simulink model "PLL_Sim_Rev0"  (R2019b)
settings: Solver=VariableStepAuto  StartTime=0.0  StopTime=0.0005  RelTol=1e-3
libraries: msbPllFoundation x1, impairlib x1, dspsrcs4 x1
settings Model: Creator=connerhannon  LastModifiedBy=connerhannon

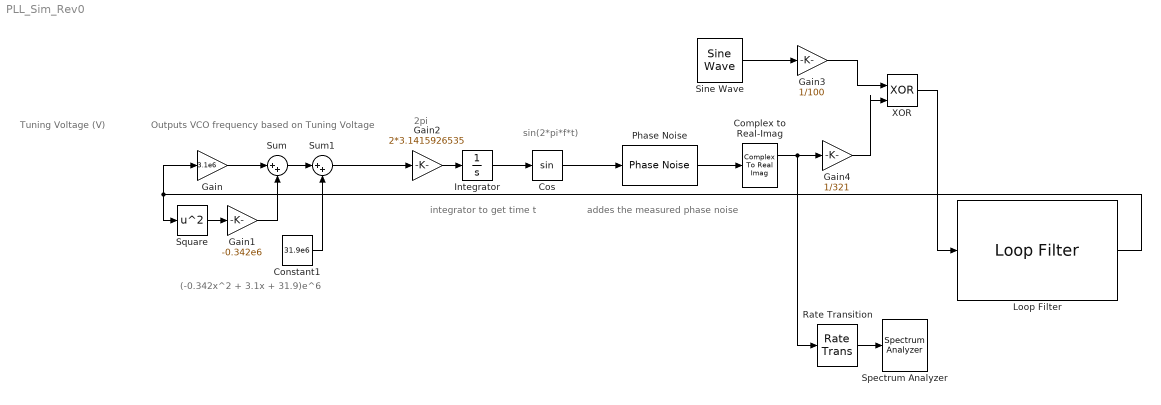
== system PLL_Sim_Rev0 ==
  note: Tuning Voltage
      | (V)
  note: 2pi
  note: sin(2*pi*f*t)
  note: integrator to get time t
  note: (-0.342x^2 + 3.1x + 31.9)e^6
  note: addes the measured phase noise
  note: Outputs VCO frequency based on Tuning Voltage
  Complex to Real-Imag : ComplexToRealImag
  Constant1 : Constant  Value=31.9e6
  Cos : Trigonometry  OutputSignalType=complex
  Gain : Gain  Gain=3.1e6
  Gain1 : Gain  Gain=-0.342e6
  Gain2 : Gain  Gain=2*3.1415926535
  Gain3 : Gain  Gain=1/100
  Gain4 : Gain  Gain=1/321
  Integrator : Integrator
  Loop Filter : msbPllFoundation/Loop Filter  FilterType="3rd  order passive"  C1=220e-12  C2=80e-9  C3=12e-12  C4=1e-12  R2=62e3  R3=1e3  R4=12e3  ExtraBuffer=off  NBuffer=1000  EnableImpairments=off  Temperature=30
      settings: SourceProductName=Mixed-Signal Blockset  SourceProductBaseCode=AM
  Phase Noise : impairlib/Phase Noise  Level=[ -36, -73, -83, -90, -112 ]  FrequencyOffset=[ 100, 400, 1000, 5000, 250000]  SampleRate=550000  RandomStream=mt19937ar with seed  Seed=1e6  SimulateUsing=Interpreted execution
      settings: SourceProductName=SerDes Toolbox  SourceProductBaseCode=SX
  Rate Transition : RateTransition  OutPortSampleTime=1/1000000000
  Sine Wave : dspsrcs4/Sine Wave  Amplitude=1  Frequency=10e6  Phase=0  SampleMode=Discrete  OutComplex=Real  CompMethod=Trigonometric fcn  TableSize=Speed  SampleTime=1/1000000  SamplesPerFrame=1  ResetState=Restart at time zero  OutputFrames=off  dataType=double  wordLen=16  udDataType=sfix(16)  fracBitsMode=Best precision  numFracBits=15  OutDataTypeStr=double  LastOutDataTypeStr=double
  Spectrum Analyzer : SpectrumAnalyzer
  Square : Math  Operator=square  SignedPower=off  SaturateOnIntegerOverflow=on
  Sum : Sum  Inputs=|++
  Sum1 : Sum  Inputs=|++
  XOR : Logic  Operator=XOR  IconShape=distinctive  AllPortsSameDT=off  OutDataTypeStr=boolean
  wires:
  Gain/1 -> Sum/1
  Sum1/1 -> Gain2/1
  Constant1/1 -> Sum1/2
  Integrator/1 -> Cos/1
  Cos/1 -> Phase Noise/1
  Phase Noise/1 -> Complex to Real-Imag/1
  Gain2/1 -> Integrator/1
  Loop Filter/1 -> Gain/1, Square/1
  Gain1/1 -> Sum/2
  Sum/1 -> Sum1/1
  Square/1 -> Gain1/1
  Complex to Real-Imag/1 -> Rate Transition/1, Gain4/1
  Sine Wave/1 -> Gain3/1
  Gain3/1 -> XOR/1
  Gain4/1 -> XOR/2
  XOR/1 -> Loop Filter/1
  Rate Transition/1 -> Spectrum Analyzer/1
